simulink model "accum_response_gold"  (R2021b)
settings: Solver=VariableStepAuto  StartTime=0.0  StopTime=6  RelTol=1e-3
undefined symbols (not defined in the file): DiscIntNeverNeededParam
libraries: simulink x1, hdlsllib x1
settings Model: Creator=hohjo  LastModifiedBy=hohjo
settings DebuggingCC: UnconnectedInputMsg=none  UnconnectedOutputMsg=none  UnconnectedLineMsg=none
settings RTWCC: DLArmComputeVersion=20.02.1

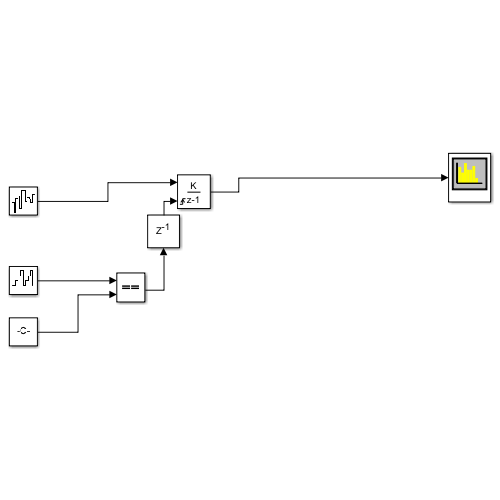
[thumbnail: Simulink's stored preview of the top-level diagram]
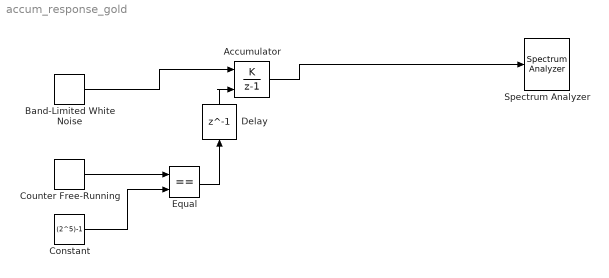
== system accum_response_gold ==
  Accumulator : DiscreteIntegrator  IntegratorMethod=Accumulation: Forward Euler  ExternalReset=rising  SampleTime=-1  ICPrevOutput=DiscIntNeverNeededParam  ICPrevScaledInput=DiscIntNeverNeededParam
  Band-Limited White Noise : simulink/Sources/Band-Limited White Noise  Cov=[0.01]  Ts=1/500000  seed=[23341]
  Constant : Constant  Value=(2^5)-1  SampleTime=1/500000
  Counter Free-Running : hdlsllib/Sources/Counter Free-Running  NumBits=5  tsamp=1/500000
      settings: SourceProductBaseCode=SL
  Delay : Delay  DelayLength=1  InitialCondition=0
  Equal : RelationalOperator  Operator===  OutDataTypeStr=boolean  RndMeth=Simplest
  Spectrum Analyzer : SpectrumAnalyzer
  wires:
  Counter Free-Running/1 -> Equal/1
  Constant/1 -> Equal/2
  Band-Limited White Noise/1 -> Accumulator/1
  Equal/1 -> Delay/1
  Delay/1 -> Accumulator/2
  Accumulator/1 -> Spectrum Analyzer/1
